simulink model "myDemo"  (R2022a)
settings: Solver=FixedStepAuto  StartTime=0.0  StopTime=1  FixedStep=0.000001  MaxStep=1e-6  RelTol=1e-3
values from neighbouring files (symbols this model uses):
  fsw = 1000000    [test.m]
  J = sum((r_interp - y_data).^2)    [test.m]
  kt = 0.137    [test.m]
  l = 1.7E-03    (= 0.0017)    [test.m]
  max_current = 2.8    [test.m]
  period_duty = 1    [test.m]
  r = 6.61    [test.m]
  rs = 0.72    [test.m]
  torque_slope = 2.646E-04    (= 0.0002646)    [test.m]
  vs = 72    [test.m]
libraries: nesl_utility x27, ee_lib x20, fl_lib x19, simulink x6, slpidlib x3
(part 2 of 2)

== system myDemo/Power Source/RMS out current ==
  input : Inport
  Display : Display
      settings: Format=short_e  Floating=on
  Gain1 : Gain  Gain=1/t
  Integrator : Integrator
  Product : Product
  Sqrt : Sqrt
  Subtract : Sum  Inputs=+-
  Transport Delay : TransportDelay  DelayTime=t
  integrating time : Constant  Value=t
  RMS : Outport
  wires:
  integrating time/1 -> ?
  Transport Delay/1 -> Subtract/2
  Integrator/1 -> Transport Delay/1, Subtract/1
  Subtract/1 -> Gain1/1
  input/1 -> Product/1, Product/2
  Product/1 -> Integrator/1
  Sqrt/1 -> RMS/1
  Gain1/1 -> Sqrt/1  "mean"
